simulink model "run_smlk"  (R2022a)
settings: Solver=ode4  StartTime=0.0  StopTime=30  FixedStep=0.01  RelTol=1e-3
values from neighbouring files (symbols this model uses):
  S = S.trimplane(xo,uo,[10])    [init_sim.m]
  ut = S.Trim.utrim    [init_sim.m]
  xt = S.Trim.xtrim    [init_sim.m]
undefined symbols (not defined in the file or in its folder): smlk_model
settings Model: Creator=danie  LastModifiedBy=danie

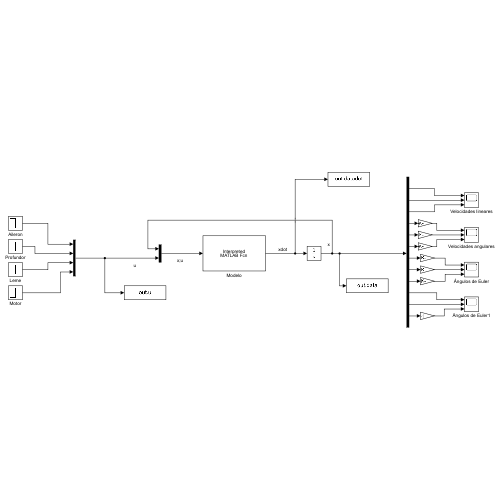
[thumbnail: Simulink's stored preview of the top-level diagram]
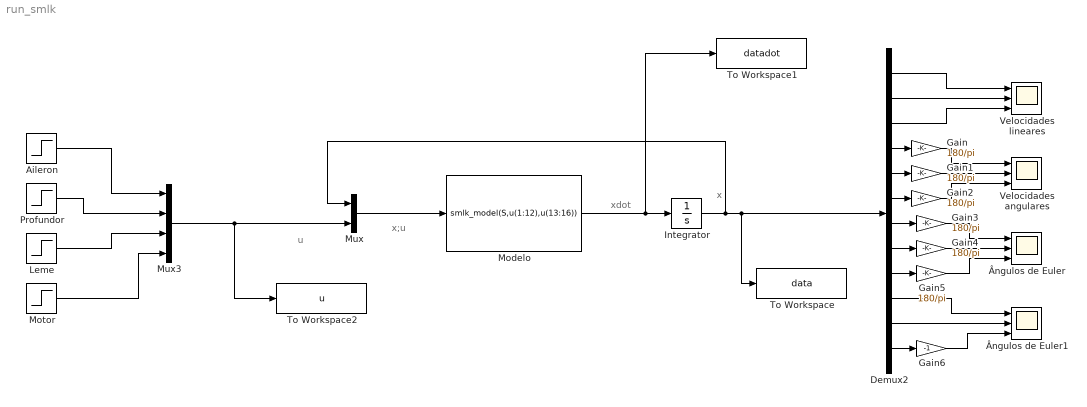
== system run_smlk ==
  note: u
  note: x;u
  note: xdot
  note: x
  Aileron : Step  Time=0  After=ut(1)  SampleTime=0
  Demux2 : Demux  Outputs=12
  Gain{,1..5} (6 alike) : Gain  Gain=180/pi
  Gain6 : Gain  Gain=-1
  Integrator : Integrator  InitialCondition=xt
  Leme : Step  Time=0  After=ut(3)  SampleTime=0
  Modelo : MATLABFcn  MATLABFcn=smlk_model(S,u(1:12),u(13:16))
  Motor : Step  Time=0  After=ut(4)  SampleTime=0
  Mux : Mux  Inputs=2
  Mux3 : Mux
  Profundor : Step  Time=0  After=ut(2)  SampleTime=0
  To Workspace : ToWorkspace  VariableName=data  SaveFormat=Timeseries  SampleTime=-1
  To Workspace1 : ToWorkspace  VariableName=datadot  SaveFormat=Timeseries  SampleTime=-1
  To Workspace2 : ToWorkspace  VariableName=u  SaveFormat=Timeseries  SampleTime=-1
  Velocidades angulares : Scope  NumInputPorts=3
  Velocidades lineares : Scope  NumInputPorts=3
  Ângulos de Euler : Scope  NumInputPorts=3
  Ângulos de Euler1 : Scope  NumInputPorts=3
  wires:
  Mux/1 -> Modelo/1
  Modelo/1 -> To Workspace1/1, Integrator/1
  Motor/1 -> Mux3/4
  Leme/1 -> Mux3/3
  Aileron/1 -> Mux3/1
  Profundor/1 -> Mux3/2
  Mux3/1 -> To Workspace2/1, Mux/2
  Integrator/1 -> To Workspace/1, Demux2/1, Mux/1
  Demux2/2 -> Velocidades lineares/2
  Demux2/1 -> Velocidades lineares/1
  Demux2/3 -> Velocidades lineares/3
  Demux2/4 -> Gain/1
  Demux2/5 -> Gain1/1
  Demux2/6 -> Gain2/1
  Gain/1 -> Velocidades angulares/1
  Gain1/1 -> Velocidades angulares/2
  Gain2/1 -> Velocidades angulares/3
  Gain5/1 -> Ângulos de Euler/3
  Gain4/1 -> Ângulos de Euler/2
  Gain3/1 -> Ângulos de Euler/1
  Demux2/7 -> Gain3/1
  Demux2/8 -> Gain4/1
  Demux2/9 -> Gain5/1
  Demux2/10 -> Ângulos de Euler1/1
  Demux2/11 -> Ângulos de Euler1/2
  Demux2/12 -> Gain6/1
  Gain6/1 -> Ângulos de Euler1/3
